simulink model "chap8_3zunaed"  (R2020a)
settings: Solver=VariableStepAuto  StartTime=0.0  StopTime=20  RelTol=1e-3
settings Model: Creator=ZUNAED  LastModifiedBy=ZUNAED

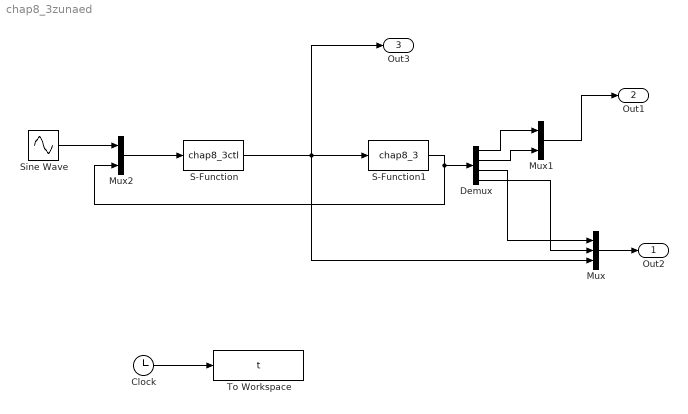
== system chap8_3zunaed ==
  Clock : Clock
  Demux : Demux
  Mux : Mux  Inputs=3
  Mux1 : Mux  Inputs=2
  Mux2 : Mux  Inputs=2
  S-Function : S-Function  FunctionName=chap8_3ctl  SFunctionDeploymentMode=off  EnableBusSupport=off
  S-Function1 : S-Function  FunctionName=chap8_3  SFunctionDeploymentMode=off  EnableBusSupport=off
  Sine Wave : Sin  SampleTime=0.001
  To Workspace : ToWorkspace  VariableName=t  SaveFormat=Timeseries  SampleTime=-1
  Out2 : Outport  SignalName=p
  Out1 : Outport  Port=2  SignalName=y
  Out3 : Outport  Port=3  SignalName=ut
  wires:
  Sine Wave/1 -> Mux2/1
  Mux2/1 -> S-Function/1
  S-Function1/1 -> Mux2/2, Demux/1
  Demux/1 -> Mux1/1
  Demux/2 -> Mux1/2
  Mux1/1 -> Out1/1
  Clock/1 -> To Workspace/1
  Demux/3 -> Mux/1
  Mux/1 -> Out2/1
  S-Function/1 -> Mux/3, Out3/1, S-Function1/1
  Demux/4 -> Mux/2
